simulink model "ASSIGNMENT2"  (R2020a)
settings: Solver=FixedStepAuto  StartTime=0.0  StopTime=10.0  FixedStep=1e-3  RelTol=1e-3  EnableMultiTasking=on
undefined symbols (not defined in the file): A0, A1, D0, D1, D10, D11, D12, D13, D2, D3, D4, D5, D6, D7, D8, D9, PTA0, PTA1, PTA2, PTB2, PTB23, PTB3, PTB9, PTC16, PTC17, PTC2, PTC3, PTC4, PTD0, PTD1, PTD2, PTD3
libraries: frdmk64flib x22, etargetslib x12
settings Model: ExtModeTrigDuration=5  Creator=nguye  LastModifiedBy=josht
settings OptimizationCC: EnhancedBackFolding=on  PassReuseOutputArgsAs=Individual arguments  ZeroExternalMemoryAtStartup=off  ZeroInternalMemoryAtStartup=off  MaxStackSize=64  OptimizeBlockOrder=speed  DifferentSizesBufferReuse=on  OptimizationCustomize=off  EfficientTunableParamExpr=on
settings DebuggingCC: ParameterTunabilityLossMsg=error
settings HardwareCC: ProdBitPerPointer=32  ProdBitPerSizeT=32  ProdBitPerPtrDiffT=32  ProdLargestAtomicInteger=Long  ProdLargestAtomicFloat=Double  ProdWordSize=32  ProdHWDeviceType=ARM Compatible->ARM Cortex
settings SFSimCC: MATLABDynamicMemAlloc=off
settings RTWCC: SystemTargetFile=ert.tlc  HardwareBoard=NXP FRDM-K64F  TemplateMakefile=ert_default_tmf  Toolchain=GNU Tools for ARM Embedded Processors
settings CodeAppCC: ForceParamTrailComments=on  IgnoreCustomStorageClasses=off  OperatorAnnotations=on  SimulinkDataObjDesc=on  SFDataObjDesc=on  InsertBlockDesc=on

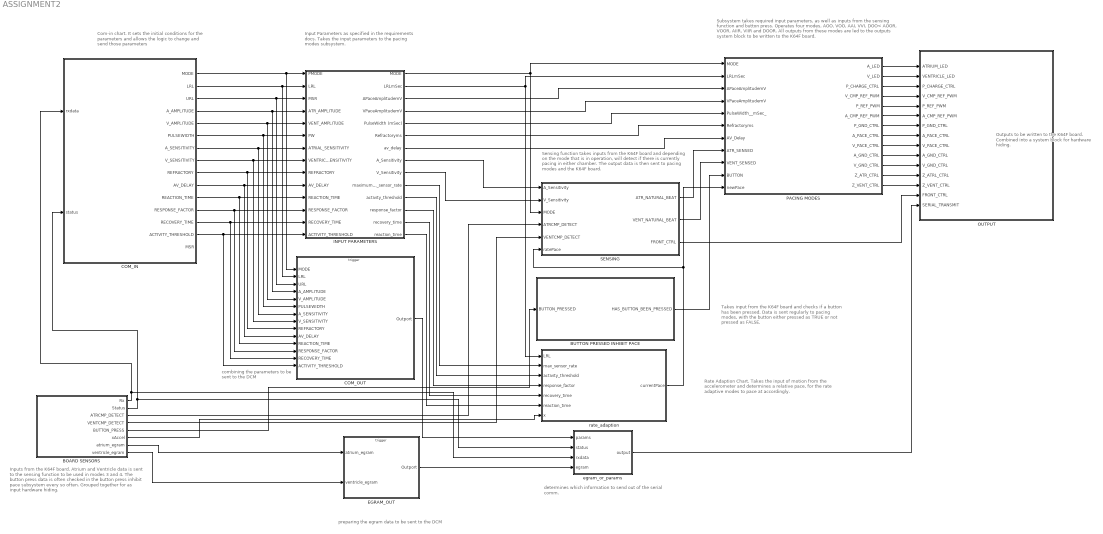
== system ASSIGNMENT2 ==
  note: Com-in chart. It sets the initial conditions for
      | the parameters and allows the logic to change
      | and send those parameters
  note: combining the parameters to be
      | sent to the DCM
  note: preparing the egram data to be sent to the DCM
  note: determines which information to send out of the serial
      | comm.
  note: Rate Adaption Chart. Takes the input of motion from the
      | accelerometer and determines a relative pace, for the rate
      | adaptive modes to pace at accordingly.
  note: Outputs to be written to the K64F board. Combined into a system block for hardware hiding.
  note: Subsystem takes required input parameters, as well as inputs from the sensing function and button press. Operates four modes, AOO, VOO, AAI, VVI, DOO< AOOR, VOOR, AIIR, VIIR and DOOR. All outputs from these modes are led to the outputs system block to be written to the K64F board.
  note: Takes input from the K64F board and checks if a button has been pressed. Data is sent regularly to pacing modes, with the button either pressed as TRUE or not pressed as FALSE.
  note: Sensing function takes inputs from the K64F board and depending on the mode that is in operation, will detect if there is currently pacing in either chamber. The output data is then sent to pacing modes and the K64F board.
  note: Inputs from the K64F board. Atrium and Ventricle data is sent to the sensing function to be used in modes 3 and 4. The button press data is often checked in the button press inhibit pace subsystem every so often. Grouped together for as input hardware hiding.
  note: Input Parameters as specified in the requirements docs. Takes the input parameters to the pacing modes subsystem.
  BOARD SENSORS : Subsystem
  BUTTON PRESSED INHIBIT PACE : Stateflow chart  TreatAsAtomicUnit=on
  COM_IN : Stateflow chart  TreatAsAtomicUnit=on
      settings: PortSchema="{\"entries\":[{\"content\":{\"sides\":[{\"content\":{\"connectorIds\":[\"In1\",\"In2\"]},\"type\":\"ConnectorPlacement.EquallySpacedRectSide\",\"uuid\":\"619e0db2-2bf7-421b-b558-4fd45d7ba277\"},{\"content\":{\"connectorIds\":[\"Out1\",\"Out2\",\"Out3\",\"Out4\",\"Out5\",\"Out6\",\"Out7\",\"Out8\",\"Out9\",\"Out10\",\"Out12\",\"Out13\",\"Out14\",\"Out11\",\"Out15\"],\"side\":\"RIGHT\"},\"type\":\"ConnectorPlacement.EquallySpacedRectSide\",\"uuid\":\"e3ef0451-1585-4711-a77b-fa2f1afc3d48\"},{\"content\":{\"connectorIds\":[],\"side\":\"TOP\"},\"type\":\"ConnectorPlacement.EquallySpacedRectSide\",\"uuid\":\"85336d80-516e-4cef-9045-d04e52d072f5\"}]},\"type\":\"ConnectorPlacement.EquallySpacedConnector\",\"uuid\":\"89f7fae5-c683-4cd3-bd83-79eb44a74088\"}],\"packageUris\":[\"http://schema.mathworks.com/mf0/Connector/19700101\"],\"version\":\"1.0\"}"
  COM_OUT : Subsystem  TreatAsAtomicUnit=on
  EGRAM_OUT : Subsystem
  INPUT PARAMETERS : Subsystem
  OUTPUT : Subsystem
  PACING MODES : Stateflow chart  TreatAsAtomicUnit=on
      settings: PortSchema="{\"entries\":[{\"content\":{\"sides\":[{\"content\":{\"connectorIds\":[\"In5\",\"In3\",\"In1\",\"In10\",\"In2\",\"In4\",\"In9\",\"In11\",\"In6\",\"In7\",\"In8\"]},\"type\":\"ConnectorPlacement.EquallySpacedRectSide\",\"uuid\":\"91d004aa-36cd-4c69-a917-f79b2844d6aa\"},{\"content\":{\"connectorIds\":[\"Out1\",\"Out2\",\"Out3\",\"Out4\",\"Out5\",\"Out6\",\"Out7\",\"Out8\",\"Out9\",\"Out10\",\"Out11\",\"Out12\",\"Out13\"],\"side\":\"RIGHT\"},\"type\":\"ConnectorPlacement.EquallySpacedRectSide\",\"uuid\":\"0665768b-03e4-4e98-bed3-39033520654e\"},{\"content\":{\"connectorIds\":[],\"side\":\"TOP\"},\"type\":\"ConnectorPlacement.EquallySpacedRectSide\",\"uuid\":\"14fb5a70-d6f2-4ae1-b3e6-093518f8f689\"}]},\"type\":\"ConnectorPlacement.EquallySpacedConnector\",\"uuid\":\"d5ca5d76-dd04-4799-9f0a-4919c9752c3c\"}],\"packageUris\":[\"http://schema.mathworks.com/mf0/Connector/19700101\"],\"version\":\"1.0\"}"
  SENSING : Stateflow chart  TreatAsAtomicUnit=on
      settings: PortSchema="{\"entries\":[{\"content\":{\"sides\":[{\"content\":{\"connectorIds\":[\"In2\",\"In1\",\"In3\",\"In4\",\"In5\",\"In6\"]},\"type\":\"ConnectorPlacement.EquallySpacedRectSide\",\"uuid\":\"bc0061e5-2268-4ed3-88e3-9935ce96967c\"},{\"content\":{\"connectorIds\":[\"Out1\",\"Out3\",\"Out2\"],\"side\":\"RIGHT\"},\"type\":\"ConnectorPlacement.EquallySpacedRectSide\",\"uuid\":\"8fba571b-2cb4-41f0-94d7-5bd4581741f0\"},{\"content\":{\"connectorIds\":[],\"side\":\"TOP\"},\"type\":\"ConnectorPlacement.EquallySpacedRectSide\",\"uuid\":\"c5b92805-16d4-4d46-b726-9ca32eadec12\"}]},\"type\":\"ConnectorPlacement.EquallySpacedConnector\",\"uuid\":\"9c7c7a33-77bb-4cd8-a2bd-d6fdb4615ef7\"}],\"packageUris\":[\"http://schema.mathworks.com/mf0/Connector/19700101\"],\"version\":\"1.0\"}"
  egram_or_params : Stateflow chart  TreatAsAtomicUnit=on
      settings: PortSchema="{\"entries\":[{\"content\":{\"sides\":[{\"content\":{\"connectorIds\":[\"In3\",\"In4\",\"In1\",\"In2\"]},\"type\":\"ConnectorPlacement.EquallySpacedRectSide\",\"uuid\":\"69dcc80b-0ea0-4d23-be0a-c51a47c20cb1\"},{\"content\":{\"connectorIds\":[\"Out1\"],\"side\":\"RIGHT\"},\"type\":\"ConnectorPlacement.EquallySpacedRectSide\",\"uuid\":\"c9fe292f-d14c-4f62-8723-6ac4ea5088e7\"},{\"content\":{\"connectorIds\":[],\"side\":\"TOP\"},\"type\":\"ConnectorPlacement.EquallySpacedRectSide\",\"uuid\":\"d77d51ee-8e15-486d-aa7f-09cbbff666ae\"}]},\"type\":\"ConnectorPlacement.EquallySpacedConnector\",\"uuid\":\"0aae601c-aac5-450b-8d5f-260899d17668\"}],\"packageUris\":[\"http://schema.mathworks.com/mf0/Connector/19700101\"],\"version\":\"1.0\"}"
  rate_adaption : Stateflow chart  TreatAsAtomicUnit=on
      settings: PortSchema="{\"entries\":[{\"content\":{\"sides\":[{\"content\":{\"connectorIds\":[\"In7\",\"In1\",\"In2\",\"In3\",\"In4\",\"In5\",\"In6\"]},\"type\":\"ConnectorPlacement.EquallySpacedRectSide\",\"uuid\":\"d2c03e42-9f21-43c9-8e8f-d101396cf9c9\"},{\"content\":{\"connectorIds\":[\"Out1\"],\"side\":\"RIGHT\"},\"type\":\"ConnectorPlacement.EquallySpacedRectSide\",\"uuid\":\"774a4d93-fecc-4a6f-bb12-fa8ca3d7c9a8\"},{\"content\":{\"connectorIds\":[],\"side\":\"TOP\"},\"type\":\"ConnectorPlacement.EquallySpacedRectSide\",\"uuid\":\"cda7523f-ed4c-4147-b27e-78fd8a73452f\"}]},\"type\":\"ConnectorPlacement.EquallySpacedConnector\",\"uuid\":\"bbb2633f-e1f0-4c8f-a814-f96cdfe19ac1\"}],\"packageUris\":[\"http://schema.mathworks.com/mf0/Connector/19700101\"],\"version\":\"1.0\"}"
  wires:
  INPUT PARAMETERS/1(MODE) -> PACING MODES/5(MODE), SENSING/3(MODE)
  PACING MODES/3(P_CHARGE_CTRL) -> OUTPUT/3(P_CHARGE_CTRL)
  PACING MODES/4(V_CMP_REF_PWM) -> OUTPUT/4(V_CMP_REF_PWM)
  PACING MODES/5(P_REF_PWM) -> OUTPUT/5(P_REF_PWM)
  PACING MODES/6(A_CMP_REF_PWM) -> OUTPUT/6(A_CMP_REF_PWM)
  PACING MODES/7(P_GND_CTRL) -> OUTPUT/7(P_GND_CTRL)
  PACING MODES/8(A_PACE_CTRL) -> OUTPUT/8(A_PACE_CTRL)
  PACING MODES/9(V_PACE_CTRL) -> OUTPUT/9(V_PACE_CTRL)
  PACING MODES/10(A_GND_CTRL) -> OUTPUT/10(A_GND_CTRL)
  PACING MODES/11(V_GND_CTRL) -> OUTPUT/11(V_GND_CTRL)
  INPUT PARAMETERS/5(PulseWidth (mSec)) -> PACING MODES/2(PulseWidth__mSec_)
  INPUT PARAMETERS/6(Refractoryms) -> PACING MODES/4(Refractoryms)
  INPUT PARAMETERS/2(LRLmSec) -> PACING MODES/3(LRLmSec), rate_adaption/7(LRL)
  INPUT PARAMETERS/8(A_Sensitivity) -> SENSING/2(A_Sensitivity)
  INPUT PARAMETERS/9(V_Sensitivity) -> SENSING/1(V_Sensitivity)
  SENSING/2(FRONT_CTRL) -> OUTPUT/14(FRONT_CTRL)
  PACING MODES/12(Z_ATR_CTRL) -> OUTPUT/12(Z_ATRL_CTRL)
  PACING MODES/13(Z_VENT_CTRL) -> OUTPUT/13(Z_VENT_CTRL)
  BUTTON PRESSED INHIBIT PACE/1(HAS_BUTTON_BEEN_PRESSED) -> PACING MODES/7(BUTTON)
  INPUT PARAMETERS/10(maximum_sensor_rate) -> rate_adaption/1(max_sensor_rate)
  INPUT PARAMETERS/14(reaction_time) -> rate_adaption/5(reaction_time)
  INPUT PARAMETERS/13(recovery_time) -> rate_adaption/4(recovery_time)
  INPUT PARAMETERS/12(response_factor) -> rate_adaption/3(response_factor)
  INPUT PARAMETERS/11(activity_threshold) -> rate_adaption/2(activity_threshold)
  rate_adaption/1(currentPace) -> SENSING/6(ratePace), PACING MODES/8(newPace)
  COM_IN/1(MODE) -> COM_OUT/1(MODE), INPUT PARAMETERS/1(PMODE)
  COM_IN/2(LRL) -> COM_OUT/2(LRL), INPUT PARAMETERS/2(LRL)
  COM_IN/3(URL) -> COM_OUT/3(URL), INPUT PARAMETERS/3(MSR)
  COM_IN/4(A_AMPLITUDE) -> COM_OUT/4(A_AMPLITUDE), INPUT PARAMETERS/4(ATR_AMPLITUDE)
  COM_IN/5(V_AMPLITUDE) -> COM_OUT/5(V_AMPLITUDE), INPUT PARAMETERS/5(VENT_AMPLITUDE)
  COM_IN/6(PULSEWIDTH) -> COM_OUT/6(PULSEWIDTH), INPUT PARAMETERS/6(PW)
  COM_IN/7(A_SENSITIVITY) -> COM_OUT/7(A_SENSITIVITY), INPUT PARAMETERS/7(ATRIAL_SENSITIVITY)
  COM_IN/8(V_SENSITIVITY) -> COM_OUT/8(V_SENSITIVITY), INPUT PARAMETERS/8(VENTRICULAR_SENSITIVITY)
  COM_IN/9(REFRACTORY) -> COM_OUT/9(REFRACTORY), INPUT PARAMETERS/9(REFRACTORY)
  COM_IN/11(ACTIVITY_THRESHOLD) -> COM_OUT/14(ACTIVITY_THRESHOLD), INPUT PARAMETERS/14(ACTIVITY_THRESHOLD)
  COM_IN/12(REACTION_TIME) -> COM_OUT/11(REACTION_TIME), INPUT PARAMETERS/11(REACTION_TIME)
  COM_IN/13(RESPONSE_FACTOR) -> COM_OUT/12(RESPONSE_FACTOR), INPUT PARAMETERS/12(RESPONSE_FACTOR)
  COM_IN/14(RECOVERY_TIME) -> COM_OUT/13(RECOVERY_TIME), INPUT PARAMETERS/13(RECOVERY_TIME)
  COM_IN/10(AV_DELAY) -> COM_OUT/10(AV_DELAY), INPUT PARAMETERS/10(AV_DELAY)
  INPUT PARAMETERS/4(VPaceAmplitudemV) -> PACING MODES/10(VPaceAmplitudemV)
  INPUT PARAMETERS/3(APaceAmplitudemV) -> PACING MODES/1(APaceAmplitudemV)
  INPUT PARAMETERS/7("av_delay ") -> PACING MODES/9(AV_Delay)
  SENSING/1(ATR_NATURAL_BEAT) -> PACING MODES/11(ATR_SENSED)
  SENSING/3(VENT_NATURAL_BEAT) -> PACING MODES/6(VENT_SENSED)
  PACING MODES/1(A_LED) -> OUTPUT/1(ATRIUM_LED)
  PACING MODES/2(V_LED) -> OUTPUT/2(VENTRICLE_LED)
  egram_or_params/1(output) -> OUTPUT/15(SERIAL_TRANSMIT)
  COM_OUT/1(Outport) -> egram_or_params/3(params)
  EGRAM_OUT/1(Outport) -> egram_or_params/2(egram)
  BOARD SENSORS/2(Status) -> egram_or_params/4(status), COM_IN/2(status)
  BOARD SENSORS/1(Rx) -> egram_or_params/1(rxdata), COM_IN/1(rxdata)
  BOARD SENSORS/3(ATRCMP_DETECT) -> SENSING/4(ATRCMP_DETECT)
  BOARD SENSORS/4(VENTCMP_DETECT) -> SENSING/5(VENTCMP_DETECT)
  BOARD SENSORS/5(BUTTON_PRESS) -> BUTTON PRESSED INHIBIT PACE/1(BUTTON_PRESSED)
  BOARD SENSORS/6(xAccel) -> rate_adaption/6(x)
  BOARD SENSORS/7(atrium_egram) -> EGRAM_OUT/1(atrium_egram)
  BOARD SENSORS/8(ventricle_egram) -> EGRAM_OUT/2(ventricle_egram)

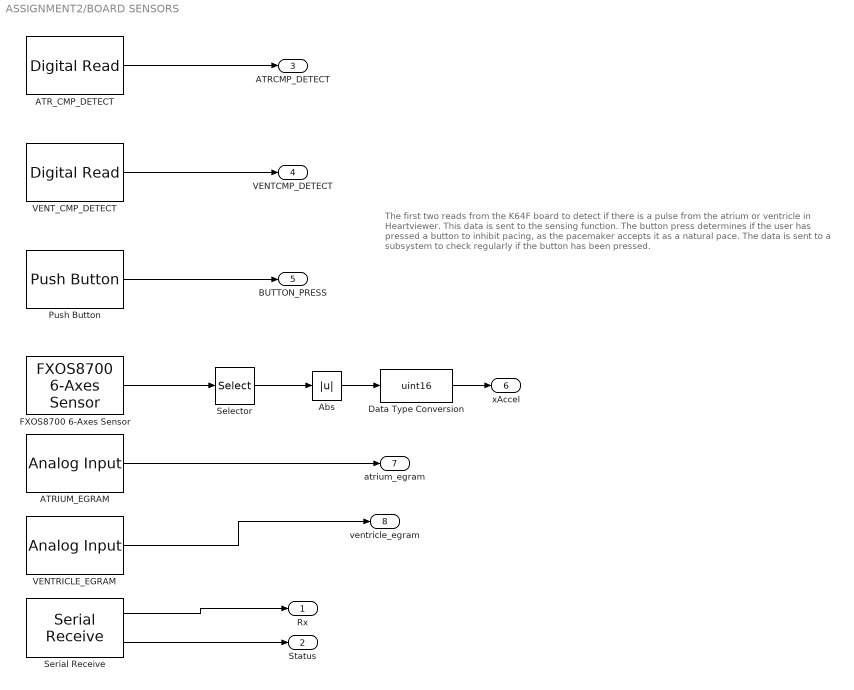
== system ASSIGNMENT2/BOARD SENSORS ==
  note: The first two reads from the K64F board to detect if there is a pulse from the atrium or ventricle in Heartviewer. This data is sent to the sensing function.
      |
      | The button press determines if the user has pressed a button to inhibit pacing, as the pacemaker accepts it as a natural pace. The data is sent to a subsystem to check regularly if the button has been pressed.
  ATRIUM_EGRAM : frdmk64flib/Analog Input  Whichpin=PTB2 (A0)  SampleTime=-1
  ATR_CMP_DETECT : frdmk64flib/Digital Read  Whichpin=PTC16 (D0)  SampleTime=-1
  Abs : Abs
  Data Type Conversion : DataTypeConversion  OutDataTypeStr=uint16
  FXOS8700 6-Axes Sensor : frdmk64flib/FXOS8700 6-Axes Sensor  Activesensor=Accelerometer only  ODR=800Hz  HybridODR=400Hz  Accelfullrange=-4g to +4g  SampleTime=-1
  Push Button : frdmk64flib/Push Button  Whichswitch=SW2  SampleTime1=-1
  Selector : Selector  InputPortWidth=3  IndexOptions=Index vector (dialog)  Indices=1  OutputSizes=1
  Serial Receive : frdmk64flib/Serial Receive  SCIModule=0  Baudrate=uint32(9600)  Parity=None  StopBits=1  HardwareFlowControl=None  ByteOrder=LittleEndian  DataType=uint8  DataLength=27  BlockingMode=off  OutputStatus=on  SampleTime=0.1
  VENTRICLE_EGRAM : frdmk64flib/Analog Input  Whichpin=PTB3 (A1)  SampleTime=-1
  VENT_CMP_DETECT : frdmk64flib/Digital Read  Whichpin=PTC17 (D1)  SampleTime=-1
  Rx : Outport
  Status : Outport  Port=2
  ATRCMP_DETECT : Outport  Port=3
  VENTCMP_DETECT : Outport  Port=4
  BUTTON_PRESS : Outport  Port=5
  xAccel : Outport  Port=6
  atrium_egram : Outport  Port=7
  ventricle_egram : Outport  Port=8
  wires:
  ATR_CMP_DETECT/1 -> ATRCMP_DETECT/1
  Push Button/1 -> BUTTON_PRESS/1
  VENT_CMP_DETECT/1 -> VENTCMP_DETECT/1
  FXOS8700 6-Axes Sensor/1 -> Selector/1
  Selector/1 -> Abs/1
  Abs/1 -> Data Type Conversion/1
  Data Type Conversion/1 -> xAccel/1
  Serial Receive/2 -> Status/1
  Serial Receive/1 -> Rx/1
  ATRIUM_EGRAM/1 -> atrium_egram/1
  VENTRICLE_EGRAM/1 -> ventricle_egram/1

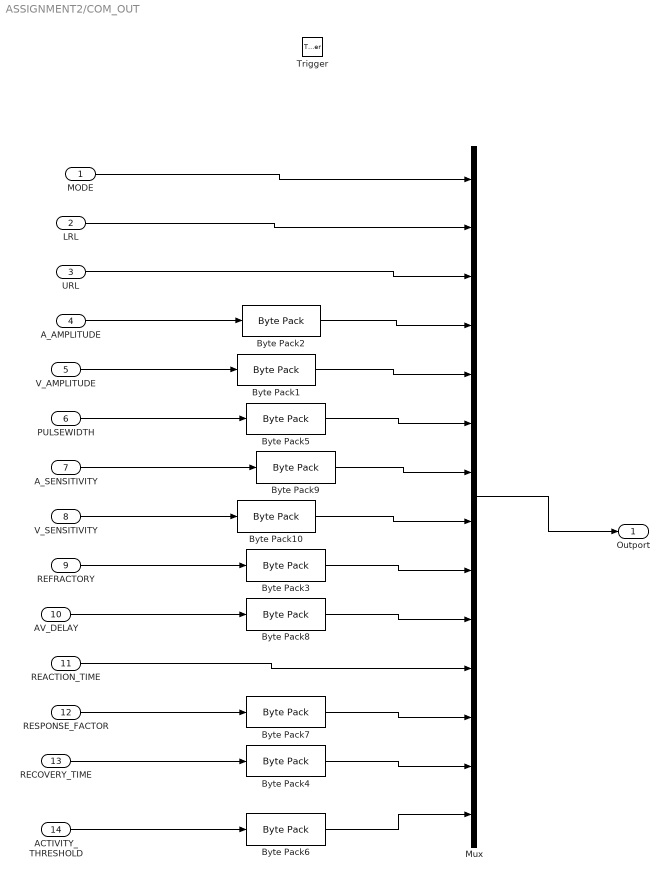
== system ASSIGNMENT2/COM_OUT ==
  MODE : Inport
  LRL : Inport  Port=2
  URL : Inport  Port=3
  A_AMPLITUDE : Inport  Port=4
  V_AMPLITUDE : Inport  Port=5
  PULSEWIDTH : Inport  Port=6
  A_SENSITIVITY : Inport  Port=7
  V_SENSITIVITY : Inport  Port=8
  REFRACTORY : Inport  Port=9
  AV_DELAY : Inport  Port=10
  REACTION_TIME : Inport  Port=11
  RESPONSE_FACTOR : Inport  Port=12
  RECOVERY_TIME : Inport  Port=13
  ACTIVITY_THRESHOLD : Inport  Port=14
  Trigger : TriggerPort  TriggerType=function-call  IsSimulinkFunction=on  FunctionName=send_params  VariantControl=Variant  PortDimensions=1
  Byte Pack{1..10} (10 alike) : etargetslib/Byte Pack  datatypes={'uint16'}  byteAlign=1
  Mux : Mux  Inputs=14
  Outport : Outport
  wires:
  MODE/1 -> Mux/1
  LRL/1 -> Mux/2
  URL/1 -> Mux/3
  A_AMPLITUDE/1 -> Byte Pack2/1
  V_AMPLITUDE/1 -> Byte Pack1/1
  Byte Pack1/1 -> Mux/5
  Byte Pack2/1 -> Mux/4
  PULSEWIDTH/1 -> Byte Pack5/1
  A_SENSITIVITY/1 -> Byte Pack9/1
  V_SENSITIVITY/1 -> Byte Pack10/1
  REFRACTORY/1 -> Byte Pack3/1
  Byte Pack3/1 -> Mux/9
  ACTIVITY_THRESHOLD/1 -> Byte Pack6/1
  REACTION_TIME/1 -> Mux/11
  RECOVERY_TIME/1 -> Byte Pack4/1
  RESPONSE_FACTOR/1 -> Byte Pack7/1
  Byte Pack5/1 -> Mux/6
  Byte Pack7/1 -> Mux/12
  Byte Pack4/1 -> Mux/13
  AV_DELAY/1 -> Byte Pack8/1
  Byte Pack9/1 -> Mux/7
  Byte Pack10/1 -> Mux/8
  Mux/1 -> Outport/1
  Byte Pack6/1 -> Mux/14
  Byte Pack8/1 -> Mux/10

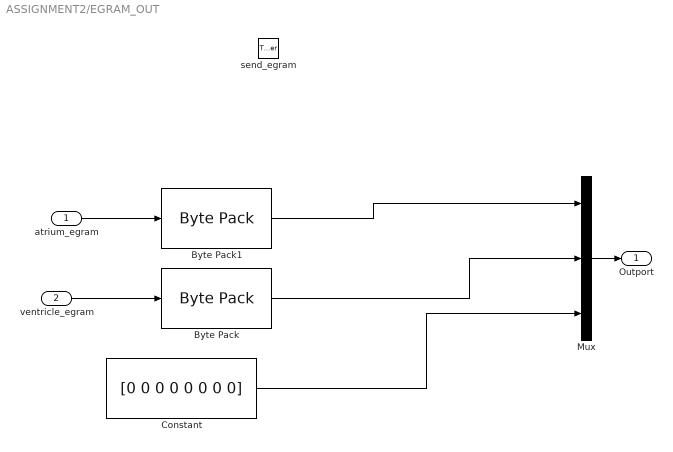
== system ASSIGNMENT2/EGRAM_OUT ==
  atrium_egram : Inport
  ventricle_egram : Inport  Port=2
  send_egram : TriggerPort  TriggerType=function-call  IsSimulinkFunction=on  FunctionName=send_egram  VariantControl=Variant  PortDimensions=1
  Byte Pack : etargetslib/Byte Pack  datatypes={'double'}  byteAlign=1
  Byte Pack1 : etargetslib/Byte Pack  datatypes={'double'}  byteAlign=1
  Constant : Constant  Value=[0 0 0 0 0 0 0 0]  OutDataTypeStr=uint8
  Mux : Mux  Inputs=3
  Outport : Outport
  wires:
  Mux/1 -> Outport/1
  ventricle_egram/1 -> Byte Pack/1
  Byte Pack/1 -> Mux/2
  Byte Pack1/1 -> Mux/1
  atrium_egram/1 -> Byte Pack1/1
  Constant/1 -> Mux/3

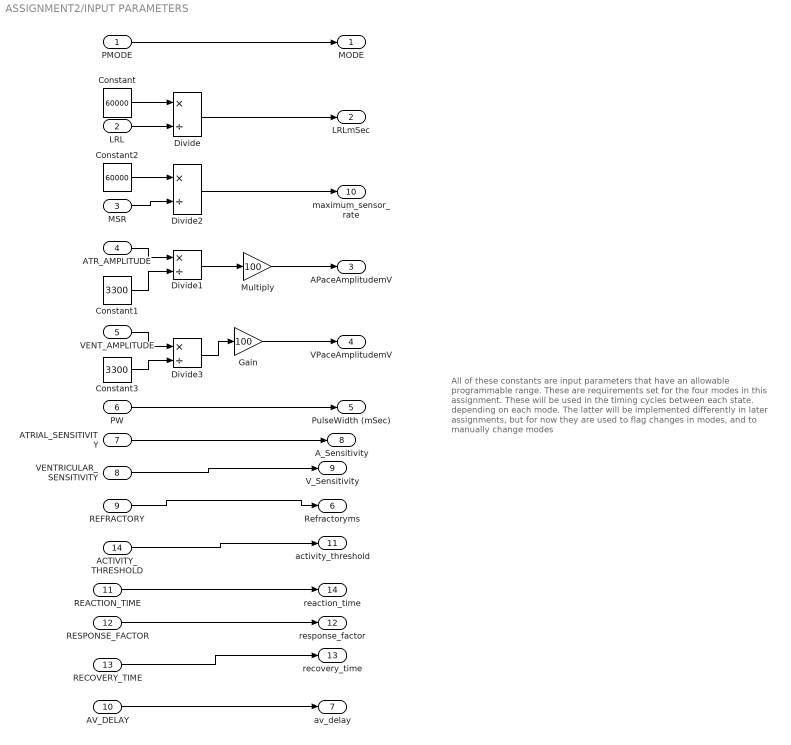
== system ASSIGNMENT2/INPUT PARAMETERS ==
  note: All of these constants are input parameters that have an allowable programmable range. These are requirements set for the four modes in this assignment. These will be used in the timing cycles between each state. depending on each mode.
      |
      | The latter will be implemented differently in later assignments, but for now they are used to flag changes in modes, and to manually change modes
  PMODE : Inport
  LRL : Inport  Port=2
  MSR : Inport  Port=3
  ATR_AMPLITUDE : Inport  Port=4
  VENT_AMPLITUDE : Inport  Port=5
  PW : Inport  Port=6
  ATRIAL_SENSITIVITY : Inport  Port=7
  VENTRICULAR_SENSITIVITY : Inport  Port=8
  REFRACTORY : Inport  Port=9
  AV_DELAY : Inport  Port=10
  REACTION_TIME : Inport  Port=11
  RESPONSE_FACTOR : Inport  Port=12
  RECOVERY_TIME : Inport  Port=13
  ACTIVITY_THRESHOLD : Inport  Port=14
  Constant : Constant  Value=60000  OutDataTypeStr=uint16
  Constant1 : Constant  Value=3300
  Constant2 : Constant  Value=60000  OutDataTypeStr=uint16
  Constant3 : Constant  Value=3300
  Divide{,1..3} (4 alike) : Product  Inputs=*/
  Gain : Gain  Gain=100
  Multiply : Gain  Gain=100
  MODE : Outport
  LRLmSec : Outport  Port=2  OutDataTypeStr=uint16
  APaceAmplitudemV : Outport  Port=3
  VPaceAmplitudemV : Outport  Port=4
  PulseWidth (mSec) : Outport  Port=5  OutDataTypeStr=uint16
  Refractoryms : Outport  Port=6
  "av_delay " : Outport  Port=7
  A_Sensitivity : Outport  Port=8
  V_Sensitivity : Outport  Port=9
  maximum_sensor_rate : Outport  Port=10  OutDataTypeStr=uint16
  activity_threshold : Outport  Port=11
  response_factor : Outport  Port=12
  recovery_time : Outport  Port=13
  reaction_time : Outport  Port=14
  wires:
  PW/1 -> PulseWidth (mSec)/1
  REFRACTORY/1 -> Refractoryms/1
  VENTRICULAR_SENSITIVITY/1 -> V_Sensitivity/1
  ATRIAL_SENSITIVITY/1 -> A_Sensitivity/1
  Divide/1 -> LRLmSec/1
  PMODE/1 -> MODE/1
  ATR_AMPLITUDE/1 -> Divide1/1
  Constant1/1 -> Divide1/2
  Divide1/1 -> Multiply/1
  Multiply/1 -> APaceAmplitudemV/1
  RECOVERY_TIME/1 -> recovery_time/1
  RESPONSE_FACTOR/1 -> response_factor/1
  REACTION_TIME/1 -> reaction_time/1
  ACTIVITY_THRESHOLD/1 -> activity_threshold/1
  LRL/1 -> Divide/2
  Constant/1 -> Divide/1
  MSR/1 -> Divide2/2
  Constant2/1 -> Divide2/1
  Divide2/1 -> maximum_sensor_rate/1
  Gain/1 -> VPaceAmplitudemV/1
  Divide3/1 -> Gain/1
  Constant3/1 -> Divide3/2
  VENT_AMPLITUDE/1 -> Divide3/1
  AV_DELAY/1 -> "av_delay "/1

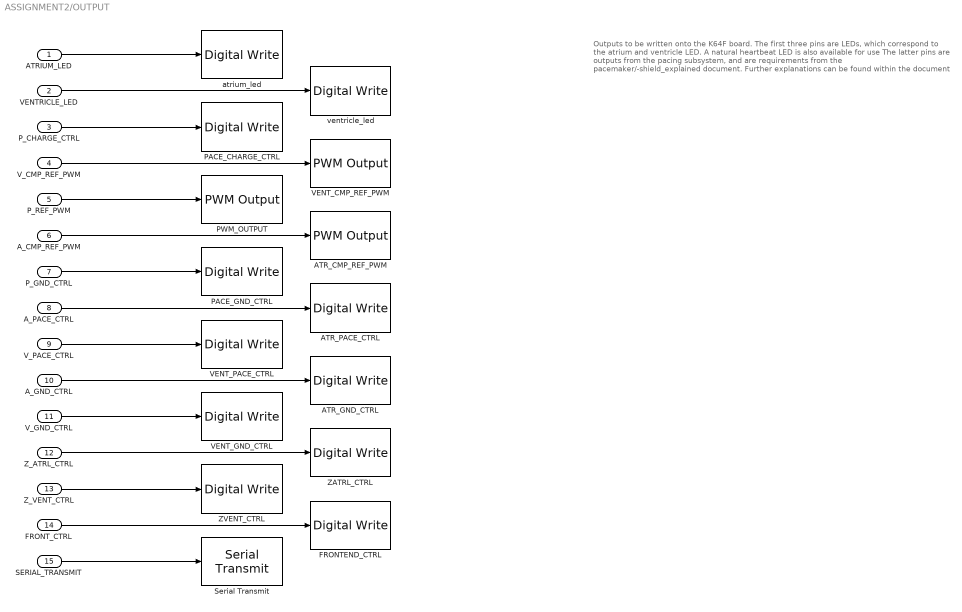
== system ASSIGNMENT2/OUTPUT ==
  note: Outputs to be written onto the K64F board.
      |
      | The first three pins are LEDs, which correspond to the atrium and ventricle LED. A natural heartbeat LED is also available for use
      |
      |
      | The latter pins are outputs from the pacing subsystem, and are requirements from the pacemaker/-shield_explained document. Further explanations can be found within the document
  ATRIUM_LED : Inport
  VENTRICLE_LED : Inport  Port=2
  P_CHARGE_CTRL : Inport  Port=3
  V_CMP_REF_PWM : Inport  Port=4
  P_REF_PWM : Inport  Port=5
  A_CMP_REF_PWM : Inport  Port=6
  P_GND_CTRL : Inport  Port=7
  A_PACE_CTRL : Inport  Port=8
  V_PACE_CTRL : Inport  Port=9
  A_GND_CTRL : Inport  Port=10
  V_GND_CTRL : Inport  Port=11
  Z_ATRL_CTRL : Inport  Port=12
  Z_VENT_CTRL : Inport  Port=13
  FRONT_CTRL : Inport  Port=14
  SERIAL_TRANSMIT : Inport  Port=15
  ATR_CMP_REF_PWM : frdmk64flib/PWM Output  Whichpin=PTC2 (D6)  InitialFrequency=2000  InitialDutyCycle=100
  ATR_GND_CTRL : frdmk64flib/Digital Write  Whichpin=PTD2 (D11)
  ATR_PACE_CTRL : frdmk64flib/Digital Write  Whichpin=PTA0 (D8)
  FRONTEND_CTRL : frdmk64flib/Digital Write  Whichpin=PTD1 (D13)
  PACE_CHARGE_CTRL : frdmk64flib/Digital Write  Whichpin=PTB9 (D2)
  PACE_GND_CTRL : frdmk64flib/Digital Write  Whichpin=PTD0 (D10)
  PWM_OUTPUT : frdmk64flib/PWM Output  Whichpin=PTA2 (D5)  InitialFrequency=2000  InitialDutyCycle=100
  Serial Transmit : frdmk64flib/Serial Transmit  SCIModule=0  Baudrate=uint32(9600)  Parity=None  StopBits=1  HardwareFlowControl=None  ByteOrder=LittleEndian  BlockingMode=on  OutputStatus=off
  VENT_CMP_REF_PWM : frdmk64flib/PWM Output  Whichpin=PTA1 (D3)  InitialFrequency=2000  InitialDutyCycle=100
  VENT_GND_CTRL : frdmk64flib/Digital Write  Whichpin=PTD3 (D12)
  VENT_PACE_CTRL : frdmk64flib/Digital Write  Whichpin=PTC4 (D9)
  ZATRL_CTRL : frdmk64flib/Digital Write  Whichpin=PTB23 (D4)
  ZVENT_CTRL : frdmk64flib/Digital Write  Whichpin=PTC3 (D7)
  atrium_led : frdmk64flib/Digital Write  Whichpin=RED_LED
  ventricle_led : frdmk64flib/Digital Write  Whichpin=GREEN_LED
  wires:
  ATRIUM_LED/1 -> atrium_led/1
  VENTRICLE_LED/1 -> ventricle_led/1
  P_CHARGE_CTRL/1 -> PACE_CHARGE_CTRL/1
  V_CMP_REF_PWM/1 -> VENT_CMP_REF_PWM/1
  P_REF_PWM/1 -> PWM_OUTPUT/1
  A_CMP_REF_PWM/1 -> ATR_CMP_REF_PWM/1
  P_GND_CTRL/1 -> PACE_GND_CTRL/1
  FRONT_CTRL/1 -> FRONTEND_CTRL/1
  A_PACE_CTRL/1 -> ATR_PACE_CTRL/1
  A_GND_CTRL/1 -> ATR_GND_CTRL/1
  V_PACE_CTRL/1 -> VENT_PACE_CTRL/1
  V_GND_CTRL/1 -> VENT_GND_CTRL/1
  Z_ATRL_CTRL/1 -> ZATRL_CTRL/1
  Z_VENT_CTRL/1 -> ZVENT_CTRL/1
  SERIAL_TRANSMIT/1 -> Serial Transmit/1

== stateflow chart ASSIGNMENT2/SENSING ==
  state LOAD_DATA
    entry:
    FRONT_CTRL = true;
  state IS_THERE_NATURAL_PACE
    entry:
    ATR_NATURAL_BEAT = false;
    VENT_NATURAL_BEAT = false;
  state VENTRICLE_SENSED
    entry:
    VENT_NATURAL_BEAT = true;
  state ATRIUM_SENSED
    entry:
    ATR_NATURAL_BEAT = true;
  note: Within the sensing function, we start off with a default tranition leading to a state that lets the board know that we are sensing.
      |
      | This leads to the next state which checks if there is a natural pace from the atrium or ventricle. In mode 3, we are testing AAI pacing,
      | and with the input from the K64F board, if there is a natural pace, the data is sent to the pacing subsystem.
      | Otherwise, the loop starts over. This works the same for mode 4, which is VVI.
  (default) -> LOAD_DATA
  LOAD_DATA -> IS_THERE_NATURAL_PACE
  (junction 56) -> IS_THERE_NATURAL_PACE [order 2] : [ATRCMP_DETECT == false]
  (junction 51) -> IS_THERE_NATURAL_PACE [order 1] : [VENTCMP_DETECT == false]
  (junction 56) -> ATRIUM_SENSED [order 1] : [ATRCMP_DETECT == true]
  IS_THERE_NATURAL_PACE -> ATRIUM_SENSED [order 2] : [ATRCMP_DETECT == true]
  IS_THERE_NATURAL_PACE -> VENTRICLE_SENSED [order 1] : [VENTCMP_DETECT == true]
  ATRIUM_SENSED -> (junction 56) : [after(ratePace,msec) || ATRCMP_DETECT == true]
  (junction 51) -> VENTRICLE_SENSED [order 2] : [VENTCMP_DETECT == true]
  VENTRICLE_SENSED -> (junction 51) : [after(ratePace,msec)||VENTCMP_DETECT == true]
  data: V_Sensitivity input; A_Sensitivity input; MODE input; ATRCMP_DETECT input; VENTCMP_DETECT input; ATR_NATURAL_BEAT output; FRONT_CTRL output; ratePace input; VENT_NATURAL_BEAT output

== stateflow chart ASSIGNMENT2/COM_IN ==
  settings: executeAtInitialization=1
  state SET_PARAM
    entry:
    MODE = rxdata(3);
    LRL = rxdata(4);
    URL = rxdata(5);
    A_AMPLITUDE = typecast(rxdata(6:7), 'uint16');
    V_AMPLITUDE = typecast(rxdata(8:9), 'uint16');
    PULSEWIDTH = typecast(rxdata(10:11), 'uint16');
    A_SENSITIVITY = typecast(rxdata(12:13), 'uint16');
    V_SENSITIVITY = typecast(rxdata(14:15), 'uint16');
    REFRACTORY = typecast(rxdata(16:17), 'uint16');
    AV_DELAY = typecast(rxdata(18:19), 'uint16');
    ACTIVITY_THRESHOLD =typecast(rxdata(20:21), 'uint16');
    REACTION_TIME = rxdata(22);
    RESPONSE_FACTOR = typecast(rxdata(23:24), 'uint16');
    RECOVERY_TIME = typecast(rxdata(25:26), 'uint16');
    MSR = rxdata(27)
  state INITIAL
    entry:
    MODE = 2;           %1-10
    LRL = 60;          %BPM
    URL = 120;        %BPM
    A_AMPLITUDE = 2000;  %mV
    V_AMPLITUDE = 2000;  %mV
    PULSEWIDTH = 1;   %msec
    A_SENSITIVITY = 3000;
    V_SENSITIVITY = 3000;
    REFRACTORY = 320;     %msec
    AV_DELAY = 100;   %msec
    ACTIVITY_THRESHOLD = 4      %1-7
    REACTION_TIME = 30;           %sec
    RESPONSE_FACTOR = 8;   %1-16
    RECOVERY_TIME = 300;      %sec
    MSR = 120;    %BPM
  state SEND_EGRAM
    entry:
    send_egram()
  state STANDBY
  state ECHO_PARAM
    entry:
    send_params();
  SEND_EGRAM -> STANDBY : [rxdata(2) == hex2dec('62')]
  (default) -> INITIAL
  SET_PARAM -> STANDBY
  (junction 11) -> SET_PARAM [order 1] : [rxdata(2) == hex2dec('55')]
  (junction 9) -> STANDBY [order 2]
  (junction 11) -> SEND_EGRAM [order 3] : [rxdata(2) == hex2dec('47')]
  INITIAL -> STANDBY
  STANDBY -> (junction 9) : [status == 0]
  (junction 9) -> (junction 11) [order 1] : [rxdata(1) == hex2dec('16')]
  (junction 11) -> ECHO_PARAM [order 2] : [rxdata(2) == hex2dec('22')]
  ECHO_PARAM -> STANDBY
  data: rxdata input uint8; status input uint8; MODE output uint8; LRL output uint8; URL output uint8; A_AMPLITUDE output uint16; V_AMPLITUDE output uint16; PULSEWIDTH output uint16; A_SENSITIVITY output uint16; V_SENSITIVITY output uint16; REFRACTORY output uint16; AV_DELAY output uint16; ACTIVITY_THRESHOLD output uint16; REACTION_TIME output uint8; RESPONSE_FACTOR output uint16; RECOVERY_TIME output uint16; MSR output uint8

== stateflow chart ASSIGNMENT2/PACING MODES ==
  settings: executeAtInitialization=1
  state V00
    note: Asynchronous Ventricular pacing in a single chamber.
        |
        | First the primary capacitor is charged and after the
        | condition statement, the ventricle is paced. The blocking
        | capacitor is then discharged and the cycle continues.
    state Charging_C22
      entry:
      A_PACE_CTRL = 0;
      V_PACE_CTRL = 0;
      P_REF_PWM = VPaceAmplitudemV;
      P_CHARGE_CTRL = 1;
      V_LED = 0;
    state PULSING1
      entry:
      P_CHARGE_CTRL = 0;
      P_GND_CTRL = 1;
      A_PACE_CTRL = 0;
      A_GND_CTRL = 0;
      Z_ATR_CTRL = 0;
      Z_VENT_CTRL = 0;
      V_GND_CTRL = 0;
      V_PACE_CTRL = 1;
      V_LED = 1;
    state DISCHARGING_BLOCKING_CAPACITOR
      entry:
      P_GND_CTRL = 1;
      V_PACE_CTRL = 0;
      Z_ATR_CTRL = 0;
      Z_VENT_CTRL = 0;
      A_PACE_CTRL = 0;
      A_GND_CTRL = 0;
      V_GND_CTRL = 1;
      V_LED = 0;
    (default) -> V00.Charging_C22
    V00.DISCHARGING_BLOCKING_CAPACITOR -> V00.Charging_C22 [order 1] : [after(Refractoryms,msec) && MODE==2]
    V00.Charging_C22 -> V00.PULSING1 : [after((LRLmSec-PulseWidth__mSec_-Refractoryms),msec)]
    V00.PULSING1 -> V00.DISCHARGING_BLOCKING_CAPACITOR : [after(PulseWidth__mSec_,msec)]
  state A00
    note: AAO mode, or Asynchronous atrial pacing.
        |
        | First we charge the primary capacitor C22 with the
        | corresponsind pin arrangement as specified in
        | requirements. After the specified amount of time in as per
        | the condition, the atrium is paced, and the blocking capacitor
        | is then discharged. The cycle continues.
    state Charging_C22
      entry:
      A_PACE_CTRL = 0;
      V_PACE_CTRL = 0;
      P_REF_PWM = APaceAmplitudemV;
      P_CHARGE_CTRL = 1;
      A_LED = 0;
    state PULSING1
      entry:
      P_CHARGE_CTRL = 0;
      P_GND_CTRL = 1;
      V_PACE_CTRL = 0;
      V_GND_CTRL = 0;
      Z_VENT_CTRL = 0;
      Z_ATR_CTRL = 0;
      A_GND_CTRL = 0;
      A_PACE_CTRL = 1;
      A_LED = 1;
    state DISCHARGING_BLOCKING_CAPACITOR
      entry:
      P_GND_CTRL = 1;
      A_PACE_CTRL = 0;
      Z_VENT_CTRL = 0;
      Z_ATR_CTRL = 0;
      V_PACE_CTRL = 0;
      V_GND_CTRL = 0;
      A_GND_CTRL = 1;
      A_LED = 0;
    A00.Charging_C22 -> A00.PULSING1 : [after((LRLmSec-PulseWidth__mSec_-Refractoryms),msec)]
    (default) -> A00.Charging_C22
    A00.DISCHARGING_BLOCKING_CAPACITOR -> A00.Charging_C22 [order 1] : [after(Refractoryms,msec) && MODE==1]
    A00.PULSING1 -> A00.DISCHARGING_BLOCKING_CAPACITOR : [after(PulseWidth__mSec_,msec)]
  state AAI
    note: Pacing mode AAI is similar to AOO with the
        | addition of a sensing function. The inputs
        | of the sensing fucntion are incorporated
        | within the conditions for the pacemaker
        | to pace appropriately. It will pace if there is
        | no natural pulse sensed. Hysterisis pacing
        | is also involved with AAI pacing as shown
        | below.
    state Charging_C22
      entry:
      A_PACE_CTRL = 0;
      V_PACE_CTRL = 0;
      P_REF_PWM = APaceAmplitudemV;
      P_CHARGE_CTRL = 1;
      A_LED = 0;
    state PULSING
      entry:
      P_CHARGE_CTRL = 0;
      P_GND_CTRL = 1;
      V_PACE_CTRL = 0;
      V_GND_CTRL = 0;
      Z_ATR_CTRL = 0;
      Z_VENT_CTRL = 0;
      A_GND_CTRL = 0;
      A_PACE_CTRL = 1;
      A_LED = 1;
    state DISCHARGING_BLOCKING_CAPACITOR
      entry:
      P_GND_CTRL = 1;
      A_PACE_CTRL = 0;
      Z_ATR_CTRL = 0;
      Z_VENT_CTRL = 0;
      V_PACE_CTRL = 0;
      V_GND_CTRL = 0;
      A_GND_CTRL = 1;
      A_LED = 0;
    (default) -> AAI.Charging_C22
    AAI.Charging_C22 -> AAI.PULSING : [after((LRLmSec-PulseWidth__mSec_-Refractoryms),msec)]
    (junction 166) -> AAI.Charging_C22 : [after(Refractoryms,msec)]
    (junction 161) -> AAI.Charging_C22 : [after(Refractoryms, msec)]
    (junction 164) -> (junction 166) : [ATR_SENSED == false]
    (junction 159) -> (junction 161) [order 1] : [ATR_SENSED == false]
    AAI.PULSING -> AAI.DISCHARGING_BLOCKING_CAPACITOR : [after(PulseWidth__mSec_,msec)]
    (junction 159) -> (junction 164) [order 2] : [ATR_SENSED == true]
    AAI.DISCHARGING_BLOCKING_CAPACITOR -> (junction 159) [order 1] : [BUTTON == false && MODE==3]
  state VVI
    note: The process behind VVI is similar to VOO, except there is
        | a sensing function involved. If a natural pace is sensed, then
        | as per the confitions in the diagram, there will be no pulse
        | from the pacemaker. If there is no natural pace sensed,
        | there will be a pulse. Hysterisis pacing is also involved
        | within VVI pacing as shown below.
    state Charging_C22
      entry:
      A_PACE_CTRL = 0;
      V_PACE_CTRL = 0;
      P_REF_PWM = VPaceAmplitudemV;
      P_CHARGE_CTRL = 1;
      V_LED = 0;
    state PULSING
      entry:
      P_CHARGE_CTRL = 0;
      P_GND_CTRL = 1;
      A_PACE_CTRL = 0;
      A_GND_CTRL = 0;
      Z_ATR_CTRL = 0;
      Z_VENT_CTRL = 0;
      V_GND_CTRL = 0;
      V_PACE_CTRL = 1;
      V_LED = 1;
    state DISCHARGING_BLOCKING_CAPACITOR
      entry:
      P_GND_CTRL = 1;
      V_PACE_CTRL = 0;
      Z_ATR_CTRL = 0;
      Z_VENT_CTRL = 0;
      A_PACE_CTRL = 0;
      A_GND_CTRL = 0;
      V_GND_CTRL = 1;
      V_LED = 0;
    (junction 156) -> VVI.Charging_C22 : [after(Refractoryms,msec)]
    (junction 154) -> (junction 156) : [VENT_SENSED == false]
    (junction 147) -> (junction 154) [order 2] : [VENT_SENSED == true]
    (junction 152) -> VVI.Charging_C22 : [after(Refractoryms,msec)]
    (default) -> VVI.Charging_C22
    (junction 147) -> (junction 152) [order 1] : [VENT_SENSED == false]
    VVI.DISCHARGING_BLOCKING_CAPACITOR -> (junction 147) [order 1] : [BUTTON == false && MODE == 4]
    VVI.Charging_C22 -> VVI.PULSING : [after((LRLmSec-PulseWidth__mSec_-Refractoryms),msec)]
    VVI.PULSING -> VVI.DISCHARGING_BLOCKING_CAPACITOR : [after(PulseWidth__mSec_,msec)]
  state START1
    entry:
    A_LED = 0;
    V_LED = 0;
    V_CMP_REF_PWM = 80;
    A_CMP_REF_PWM = 80;
  state DOO
    state Charging_V1
      entry:
      A_PACE_CTRL = 0;
      V_PACE_CTRL = 0;
      P_REF_PWM = VPaceAmplitudemV;
      P_CHARGE_CTRL = 1;
      A_LED = 0;
      %%
    state Charging_A1
      entry:
      A_PACE_CTRL = 0;
      V_PACE_CTRL = 0;
      P_REF_PWM = APaceAmplitudemV;
      P_CHARGE_CTRL = 1;
      V_LED = 0;
      %%
    state PULSING_A
      entry:
      P_CHARGE_CTRL = 0;
      P_GND_CTRL = 1;
      V_PACE_CTRL = 0;
      V_GND_CTRL = 0;
      Z_ATR_CTRL = 0;
      A_PACE_CTRL = 1;
      A_GND_CTRL = 0;
      A_LED = 1;
    note: DOO allows for all the both the atrium and ventricle to pace
        | almost simultaneously. They have to charge and discharge at a separated
        | interval called the AV_DELAY. This is a defining feature for the mode.
    state DISCHARGING_V
      entry:
      %P_CHARGE_CTRL = 0;
      V_PACE_CTRL = 0;
      Z_ATR_CTRL = 0;
      Z_VENT_CTRL = 0;
      A_PACE_CTRL = 0;
      A_GND_CTRL = 0;
      V_GND_CTRL = 1;
      V_LED = 0;
    state DISCHARGING_A
      entry:
      %P_CHARGE_CTRL = 0;
      A_PACE_CTRL = 0;
      Z_ATR_CTRL = 0;
      Z_VENT_CTRL = 0;
      V_PACE_CTRL = 0;
      V_GND_CTRL = 0;
      A_GND_CTRL = 1;
      A_LED = 0;
    state PULSING_V1
      entry:
      P_CHARGE_CTRL = 0;
      P_GND_CTRL = 1;
      A_PACE_CTRL = 0;
      A_GND_CTRL = 0;
      Z_ATR_CTRL = 0;
      Z_VENT_CTRL = 0;
      V_PACE_CTRL = 1;
      V_GND_CTRL = 0;
      V_LED = 1;
    (default) -> DOO.Charging_A1
    DOO.Charging_V1 -> DOO.PULSING_A : [after(LRLmSec - 2*AV_Delay - PulseWidth__mSec_ - Refractoryms,msec)]
    DOO.Charging_A1 -> DOO.Charging_V1 : [AV_Delay]
    DOO.DISCHARGING_V -> DOO.Charging_A1 [order 1] : [after(Refractoryms,msec) && MODE == 5]
    DOO.PULSING_A -> DOO.DISCHARGING_A : [after(PulseWidth__mSec_,msec)]
    DOO.PULSING_V1 -> DOO.DISCHARGING_V : [after(PulseWidth__mSec_,msec)]
    DOO.DISCHARGING_A -> DOO.PULSING_V1 : [after(AV_Delay - PulseWidth__mSec_,msec)]
  state A00R
    state Charging_C22
      entry:
      A_PACE_CTRL = 0;
      V_PACE_CTRL = 0;
      P_REF_PWM = APaceAmplitudemV;
      P_CHARGE_CTRL = 1;
      A_LED = 0;
    note: AOOR mode.
        |
        | Similar functionality to AOO,
        | except when movement occurs
        | the pacemaker must respond
        | with a higher designated
        | heart rate. newPace represents
        | ever-changing pace.
    state PULSING1
      entry:
      P_CHARGE_CTRL = 0;
      P_GND_CTRL = 1;
      V_PACE_CTRL = 0;
      V_GND_CTRL = 0;
      Z_ATR_CTRL = 0;
      Z_VENT_CTRL = 0;
      A_GND_CTRL = 0;
      A_PACE_CTRL = 1;
      A_LED = 1;
    state DISCHARGING_BLOCKING_CAPACITOR
      entry:
      P_GND_CTRL = 1;
      A_PACE_CTRL = 0;
      Z_ATR_CTRL = 0;
      V_PACE_CTRL = 0;
      V_GND_CTRL = 0;
      A_GND_CTRL = 1;
      A_LED = 0;
    A00R.Charging_C22 -> A00R.PULSING1 : [after((newPace-PulseWidth__mSec_-Refractoryms),msec)]
    (default) -> A00R.Charging_C22
    A00R.DISCHARGING_BLOCKING_CAPACITOR -> A00R.Charging_C22 [order 1] : [after(Refractoryms,msec) && MODE==6]
    A00R.PULSING1 -> A00R.DISCHARGING_BLOCKING_CAPACITOR : [after(PulseWidth__mSec_,msec)]
  note: Modes
      |
      | 1 - A00
      | 2 - V00
      | 3 - AAI
      | 4-  VVI
      | 5- DOOR (ASSIGNMENT 2)
      | 6 - AOOR (ASSIGNMENT 2)
      | 7 - VOOR (ASSIGNMENT 2)
      | 8 - AAIR (ASSIGNMENT 2)
      | 9 - VVIR (ASSIGNMENT 2)
      | 10 - DOOR (ASSIGNMENT 2)
      | 11 - DDDR (BONUS)
  state VOOR
    state Charging_C22
      entry:
      A_PACE_CTRL = 0;
      V_PACE_CTRL = 0;
      P_REF_PWM = VPaceAmplitudemV;
      P_CHARGE_CTRL = 1;
      V_LED = 0;
    state PULSING1
      entry:
      P_CHARGE_CTRL = 0;
      P_GND_CTRL = 1;
      A_PACE_CTRL = 0;
      A_GND_CTRL = 0;
      Z_ATR_CTRL = 0;
      Z_VENT_CTRL = 0;
      V_GND_CTRL = 0;
      V_PACE_CTRL = 1;
      V_LED = 1;
    state DISCHARGING_BLOCKING_CAPACITOR
      entry:
      P_GND_CTRL = 1;
      V_PACE_CTRL = 0;
      Z_ATR_CTRL = 0;
      Z_VENT_CTRL = 0;
      A_PACE_CTRL = 0;
      A_GND_CTRL = 0;
      V_GND_CTRL = 1;
      V_LED = 0;
    note: VOOR mode.
        |
        | Similar functionality to VOO,
        | except when movement occurs
        | the pacemaker must respond
        | with a higher designated
        | heart rate. newPace represents
        | ever-changing pace.
    (default) -> VOOR.Charging_C22
    VOOR.DISCHARGING_BLOCKING_CAPACITOR -> VOOR.Charging_C22 [order 1] : [after(Refractoryms,msec) && MODE==7]
    VOOR.Charging_C22 -> VOOR.PULSING1 : [after((newPace-PulseWidth__mSec_-Refractoryms),msec)]
    VOOR.PULSING1 -> VOOR.DISCHARGING_BLOCKING_CAPACITOR : [after(PulseWidth__mSec_,msec)]
  state AAIR
    state Charging_C22
      entry:
      A_PACE_CTRL = 0;
      V_PACE_CTRL = 0;
      P_REF_PWM = APaceAmplitudemV;
      P_CHARGE_CTRL = 1;
      A_LED = 0;
    state PULSING
      entry:
      P_CHARGE_CTRL = 0;
      P_GND_CTRL = 1;
      V_PACE_CTRL = 0;
      V_GND_CTRL = 0;
      Z_ATR_CTRL = 0;
      Z_VENT_CTRL = 0;
      A_GND_CTRL = 0;
      A_PACE_CTRL = 1;
      A_LED = 1;
    note: AIIR Mode.
        | Similar to AII mode except for the rate
        | adaptive feature, which increases the heart
        | rate based on the activity level. newPace
        | represents the ever-changing pace that
        | varies based on the activity level.
    state DISCHARGING_BLOCKING_CAPACITOR
      entry:
      P_GND_CTRL = 1;
      A_PACE_CTRL = 0;
      Z_ATR_CTRL = 0;
      Z_VENT_CTRL = 0;
      V_PACE_CTRL = 0;
      V_GND_CTRL = 0;
      A_GND_CTRL = 1;
      A_LED = 0;
    AAIR.Charging_C22 -> AAIR.PULSING : [after((newPace-Refractoryms),msec)]
    (default) -> AAIR.Charging_C22
    (junction 207) -> AAIR.Charging_C22 : [after(Refractoryms,msec)]
    (junction 208) -> AAIR.Charging_C22 : [after(Refractoryms, msec)]
    AAIR.PULSING -> AAIR.DISCHARGING_BLOCKING_CAPACITOR : [after(PulseWidth__mSec_,msec)]
    (junction 210) -> (junction 208) [order 1] : [ATR_SENSED == false]
    (junction 209) -> (junction 207) : [ATR_SENSED == false]
    (junction 210) -> (junction 209) [order 2] : [ATR_SENSED == true]
    AAIR.DISCHARGING_BLOCKING_CAPACITOR -> (junction 210) [order 1] : [BUTTON == false && MODE==8]
  state DOOR
    state Charging_V1
      entry:
      A_PACE_CTRL = 0;
      V_PACE_CTRL = 0;
      P_REF_PWM = VPaceAmplitudemV;
      P_CHARGE_CTRL = 1;
      A_LED = 0;
      %%
    state Charging_A1
      entry:
      A_PACE_CTRL = 0;
      V_PACE_CTRL = 0;
      P_REF_PWM = APaceAmplitudemV;
      P_CHARGE_CTRL = 1;
      V_LED = 0;
      %%
    state PULSING_A
      entry:
      P_CHARGE_CTRL = 0;
      P_GND_CTRL = 1;
      V_PACE_CTRL = 0;
      V_GND_CTRL = 0;
      Z_ATR_CTRL = 0;
      A_PACE_CTRL = 1;
      A_GND_CTRL = 0;
      A_LED = 1;
    note: DOOR Mode
        | Similar to DOO mode except for the
        | rate adaption feature. This allows for the
        | paced rate to increase or decrease based
        | on the activity level of the body. newPace
        | represents this ever-changing desired heart
        | rate and the logic for newPace is contained
        | in the rate_adaption chart.
    state DISCHARGING_V
      entry:
      %P_CHARGE_CTRL = 0;
      V_PACE_CTRL = 0;
      Z_ATR_CTRL = 0;
      Z_VENT_CTRL = 0;
      A_PACE_CTRL = 0;
      A_GND_CTRL = 0;
      V_GND_CTRL = 1;
      V_LED = 0;
    state DISCHARGING_A
      entry:
      %P_CHARGE_CTRL = 0;
      A_PACE_CTRL = 0;
      Z_ATR_CTRL = 0;
      Z_VENT_CTRL = 0;
      V_PACE_CTRL = 0;
      V_GND_CTRL = 0;
      A_GND_CTRL = 1;
      A_LED = 0;
    state PULSING_V1
      entry:
      P_CHARGE_CTRL = 0;
      P_GND_CTRL = 1;
      A_PACE_CTRL = 0;
      A_GND_CTRL = 0;
      Z_ATR_CTRL = 0;
      Z_VENT_CTRL = 0;
      V_PACE_CTRL = 1;
      V_GND_CTRL = 0;
      V_LED = 1;
    (default) -> DOOR.Charging_A1
    DOOR.Charging_V1 -> DOOR.PULSING_A : [after(newPace - 2*AV_Delay - PulseWidth__mSec_ - Refractoryms,msec)]
    DOOR.Charging_A1 -> DOOR.Charging_V1 : [AV_Delay]
    DOOR.DISCHARGING_V -> DOOR.Charging_A1 [order 1] : [after(Refractoryms,msec) && MODE == 10]
    DOOR.PULSING_A -> DOOR.DISCHARGING_A : [after(PulseWidth__mSec_,msec)]
    DOOR.PULSING_V1 -> DOOR.DISCHARGING_V : [after(PulseWidth__mSec_,msec)]
    DOOR.DISCHARGING_A -> DOOR.PULSING_V1 : [after(AV_Delay - PulseWidth__mSec_,msec)]
  state VVIR
    note: VIIR Mode.
        | Similar to VII mode except for the rate
        | adaptive feature, which increases the heart
        | rate based on the activity level. newPace
        | represents the ever-changing pace that
        | varies based on the activity level.
    state Charging_C22
      entry:
      A_PACE_CTRL = 0;
      V_PACE_CTRL = 0;
      P_REF_PWM = VPaceAmplitudemV;
      P_CHARGE_CTRL = 1;
      V_LED = 0;
    state PULSING
      entry:
      P_CHARGE_CTRL = 0;
      P_GND_CTRL = 1;
      A_PACE_CTRL = 0;
      A_GND_CTRL = 0;
      Z_ATR_CTRL = 0;
      Z_VENT_CTRL = 0;
      V_GND_CTRL = 0;
      V_PACE_CTRL = 1;
      V_LED = 1;
    state DISCHARGING_BLOCKING_CAPACITOR
      entry:
      P_GND_CTRL = 1;
      V_PACE_CTRL = 0;
      Z_ATR_CTRL = 0;
      Z_VENT_CTRL = 0;
      A_PACE_CTRL = 0;
      A_GND_CTRL = 0;
      V_GND_CTRL = 1;
      V_LED = 0;
    (junction 226) -> VVIR.Charging_C22 : [after(Refractoryms,msec)]
    (junction 227) -> (junction 226) : [VENT_SENSED == false]
    (junction 229) -> (junction 227) [order 2] : [VENT_SENSED == true]
    (junction 228) -> VVIR.Charging_C22 : [after(Refractoryms,msec)]
    (default) -> VVIR.Charging_C22
    (junction 229) -> (junction 228) [order 1] : [VENT_SENSED == false]
    VVIR.DISCHARGING_BLOCKING_CAPACITOR -> (junction 229) [order 1] : [BUTTON == false && MODE==9]
    VVIR.Charging_C22 -> VVIR.PULSING : [after((newPace-Refractoryms),msec)]
    VVIR.PULSING -> VVIR.DISCHARGING_BLOCKING_CAPACITOR : [after(PulseWidth__mSec_,msec)]
  START1 -> V00 [order 3] : [MODE == 2]
  DOOR.DISCHARGING_V -> START1 [order 2] : [MODE ~= 10]
  AAI.DISCHARGING_BLOCKING_CAPACITOR -> START1 [order 2] : [MODE ~= 3]
  V00.DISCHARGING_BLOCKING_CAPACITOR -> START1 [order 2] : [MODE~=2]
  VVI.DISCHARGING_BLOCKING_CAPACITOR -> START1 [order 2] : [MODE ~= 4]
  VOOR.DISCHARGING_BLOCKING_CAPACITOR -> START1 [order 2] : [MODE~=7]
  DOO.DISCHARGING_V -> START1 [order 2] : [MODE ~= 5]
  VVIR.DISCHARGING_BLOCKING_CAPACITOR -> START1 [order 2] : [MODE~=9]
  AAIR.DISCHARGING_BLOCKING_CAPACITOR -> START1 [order 2] : [MODE~=8]
  A00R.DISCHARGING_BLOCKING_CAPACITOR -> START1 [order 2] : [MODE ~= 6]
  START1 -> A00 [order 1] : [MODE == 1]
  START1 -> AAI [order 4] : [MODE == 3]
  START1 -> VVI [order 2] : [MODE == 4]
  START1 -> DOO [order 9] : [MODE == 5]
  (default) -> START1
  START1 -> A00R [order 6] : [MODE==6]
  START1 -> VOOR [order 5] : [MODE==7]
  START1 -> DOOR [order 10] : [MODE==10]
  START1 -> VVIR [order 8] : [MODE==9]
  START1 -> AAIR [order 7] : [MODE==8]
  A00.DISCHARGING_BLOCKING_CAPACITOR -> START1 [order 2] : [MODE~=1]
  data: APaceAmplitudemV input; PulseWidth__mSec_ input uint16; LRLmSec input uint16; Refractoryms input; MODE input; A_LED output; V_LED output; P_CHARGE_CTRL output; V_CMP_REF_PWM output; P_REF_PWM output; A_CMP_REF_PWM output; P_GND_CTRL output; A_PACE_CTRL output; V_PACE_CTRL output; A_GND_CTRL output; V_GND_CTRL output; VENT_SENSED input; Z_ATR_CTRL output; Z_VENT_CTRL output; BUTTON input boolean; newPace input; AV_Delay input uint16; VPaceAmplitudemV input; ATR_SENSED input

== stateflow chart ASSIGNMENT2/BUTTON PRESSED INHIBIT PACE ==
  state NO_PULSE
    entry:
    HAS_BUTTON_BEEN_PRESSED = false;
  note: A quick logic implementation to check if the onboard button has been pressed by the user
  state PULSE
    entry:
    HAS_BUTTON_BEEN_PRESSED = true;
  (default) -> NO_PULSE
  (junction 24) -> NO_PULSE [order 1] : [BUTTON_PRESSED == false]
  NO_PULSE -> PULSE : [BUTTON_PRESSED == true]
  (junction 24) -> PULSE [order 2] : [BUTTON_PRESSED == true]
  PULSE -> (junction 24) : [after(1000,msec) || BUTTON_PRESSED == true]
  data: BUTTON_PRESSED input; HAS_BUTTON_BEEN_PRESSED output boolean

== stateflow chart ASSIGNMENT2/rate_adaption ==
  note: Before any motion occurs the set pace is the LRL.
  state BASE
    entry:
    currentPace = LRL
  state SLOW_DOWN
    entry:
    currentPace = currentPace + (LRL - currentPace)/10
  state DETECTED
    entry:
    paceDelta = LRL - max_sensor_rate
    xDelta = 4 - 0.3*activity_threshold
    goalPace = LRL - paceDelta*(x - 0.3*activity_threshold)*response_factor/xDelta
  note: This loop continuously decreases the pace
      | towards resting heart rate once activity has ceased.
  note: This loop allows for the
      | pace to continuously increase
      | towards the goal pace for
      | the activity.
  state SPEED_UP
    entry:
    currentPace = currentPace - (LRL - goalPace)/10
  state NOT_DETECTED
    entry:
  (default) -> BASE
  BASE -> DETECTED : [x > 0.3*activity_threshold]
  SLOW_DOWN -> (junction 68) : [after(500,msec) || x > 0.3*activity_threshold]
  NOT_DETECTED -> SLOW_DOWN : [after(recovery_time/30,sec)]
  (junction 68) -> DETECTED [order 2] : [x > 0.3*activity_threshold]
  (junction 64) -> DETECTED [order 2] : [x > 0.3*activity_threshold]
  (junction 68) -> NOT_DETECTED [order 1] : [x < 0.3*activity_threshold]
  DETECTED -> SPEED_UP : [after(reaction_time/10,sec)]
  (junction 64) -> NOT_DETECTED [order 1] : [x < 0.3*activity_threshold]
  SPEED_UP -> (junction 64) : [after(500, msec) || x > 0.3*activity_threshold]
  data: max_sensor_rate input uint16; activity_threshold input uint16; response_factor input uint16; recovery_time input uint16; reaction_time input uint8; x input uint16; currentPace output uint16; LRL input uint16; xDelta local uint16; goalPace local uint16; paceDelta local uint16

== stateflow chart ASSIGNMENT2/egram_or_params ==
  state standby
    output = [0
    0
    0
    0
    0
    0
    0
    0
    0
    0
    0
    0
    0
    0
    0
    0
    0
    0
    0
    0
    0
    0
    0
    0];
  state SEND_PARAMS
    entry:
    output = params
  state SEND_EGRAM
    entry:
    output = egram
  SEND_PARAMS -> standby
  (default) -> standby
  (junction 13) -> SEND_PARAMS [order 2] : [rxdata(2) == hex2dec('22')]
  (junction 16) -> standby [order 1]
  standby -> (junction 16) : [status==0]
  (junction 16) -> (junction 13) [order 2] : [rxdata(1)==hex2dec('16')]
  (junction 13) -> SEND_EGRAM [order 1] : [rxdata(2) == hex2dec('47')]
  SEND_EGRAM -> standby
  data: output output; rxdata input; egram input; params input; status input
